simulink model "DualViennaRECT"  (R2021b)
settings: Solver=VariableStepAuto  StartTime=0.0  StopTime=1.5  RelTol=1e-3
libraries: spsIGBTDiodeLib x25, spsCurrentMeasurementLib x6, spsMeanLib x5, spsVoltageMeasurementLib x5, spsSeriesRLCBranchLib x3, spsMutualInductanceLib x3, spsACVoltageSourceLib x3, spsRMSLib x2, simulink x2, slpidlib x1, spsTHDLib x1, spspowerguiLib x1
settings Model: SimulationMode=accelerator  Creator=abc6820292  LastModifiedBy=abc6820292

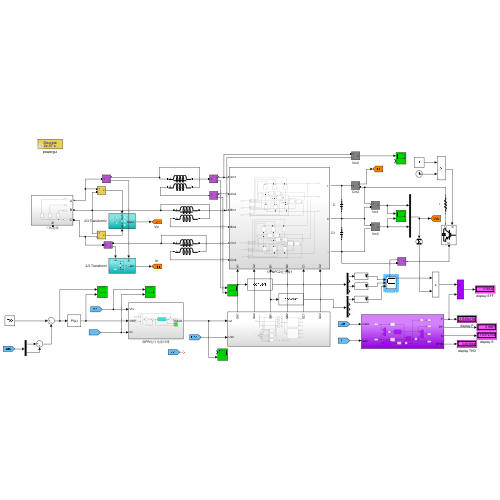
[thumbnail: Simulink's stored preview of the top-level diagram]
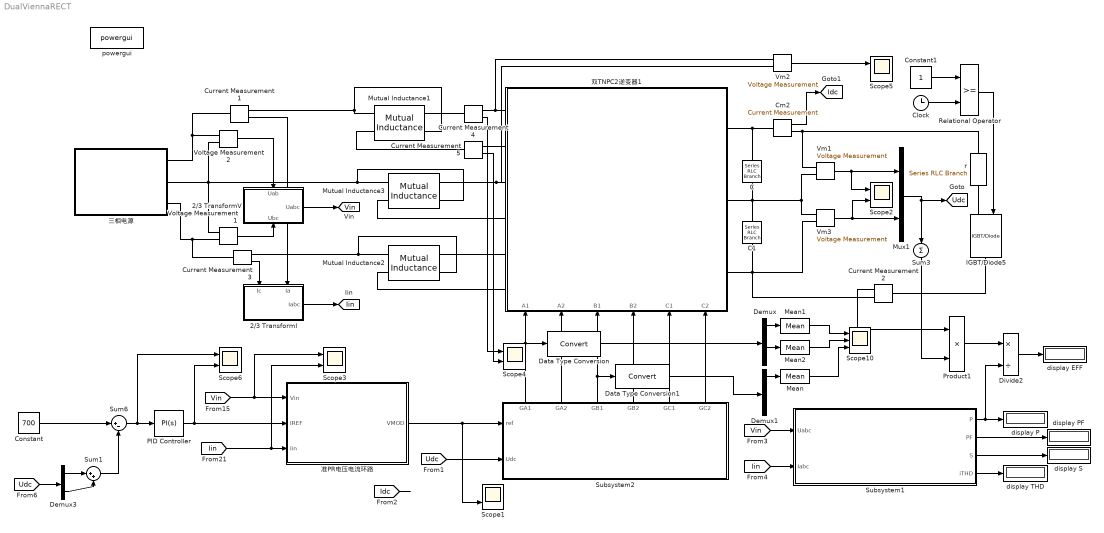
== system DualViennaRECT ==
  2/3 TransformI : Subsystem
      settings: PortSchema="{\"entries\":[{\"content\":{\"sides\":[{\"content\":{\"connectorIds\":[\"In1\",\"In2\"]},\"type\":\"ConnectorPlacement.EquallySpacedRectSide\",\"uuid\":\"58c40194-9a95-4e39-952e-f878bde7484e\"},{\"content\":{\"connectorIds\":[],\"side\":\"RIGHT\"},\"type\":\"ConnectorPlacement.EquallySpacedRectSide\",\"uuid\":\"f51692e8-3ff2-4d72-808d-3667196a4526\"},{\"content\":{\"connectorIds\":[],\"side\":\"TOP\"},\"type\":\"ConnectorPlacement.EquallySpacedRectSide\",\"uuid\":\"0aab136b-5da5-45c4-8998-999ebe8b7f2f\"},{\"content\":{\"connectorIds\":[\"Out1\"],\"side\":\"BOTTOM\"},\"type\":\"ConnectorPlacement.EquallySpacedRectSide\",\"uuid\":\"32f5f4a5-4ebb-496b-828d-b973bd46b44e\"}]},\"type\":\"ConnectorPlacement.EquallySpacedConnector\",\"uuid\":\"3ef81af7-d426-47fb-88e3-e33e58eebb83\"}],\"packageUris\":[\"http://schema.mathworks.com/mf0/Connector/R2020b\"],\"version\":\"1.0\"}"
  2/3 TransformV : Subsystem
      settings: PortSchema="{\"entries\":[{\"content\":{\"sides\":[{\"content\":{\"connectorIds\":[\"In1\"]},\"type\":\"ConnectorPlacement.EquallySpacedRectSide\",\"uuid\":\"58c40194-9a95-4e39-952e-f878bde7484e\"},{\"content\":{\"connectorIds\":[\"In2\"],\"side\":\"RIGHT\"},\"type\":\"ConnectorPlacement.EquallySpacedRectSide\",\"uuid\":\"f51692e8-3ff2-4d72-808d-3667196a4526\"},{\"content\":{\"connectorIds\":[],\"side\":\"TOP\"},\"type\":\"ConnectorPlacement.EquallySpacedRectSide\",\"uuid\":\"0aab136b-5da5-45c4-8998-999ebe8b7f2f\"},{\"content\":{\"connectorIds\":[\"Out1\"],\"side\":\"BOTTOM\"},\"type\":\"ConnectorPlacement.EquallySpacedRectSide\",\"uuid\":\"185ce796-68e2-4136-8080-97dc86d2ba54\"}]},\"type\":\"ConnectorPlacement.EquallySpacedConnector\",\"uuid\":\"3ef81af7-d426-47fb-88e3-e33e58eebb83\"}],\"packageUris\":[\"http://schema.mathworks.com/mf0/Connector/R2020b\"],\"version\":\"1.0\"}"
  C : spsSeriesRLCBranchLib/Series RLC Branch  LConnTagsString=__new0  RConnTagsString=__new0  BranchType=C  Resistance=0  Inductance=0  SetiL0=off  InitialCurrent=0  Capacitance=8e-3  Setx0=on  InitialVoltage=280  Measurements=None
  C1 : spsSeriesRLCBranchLib/Series RLC Branch  LConnTagsString=__new0  RConnTagsString=__new0  BranchType=C  Resistance=0  Inductance=0  SetiL0=off  InitialCurrent=0  Capacitance=8e-3  Setx0=on  InitialVoltage=280  Measurements=None
  Clock : Clock
  Cm2 : spsCurrentMeasurementLib/Current Measurement  PhasorSimulation=off  OutputType=Complex  PSBequivalent=0
  Constant : Constant  Value=700
  Constant1 : Constant
  Current Measurement{1..5} (5 alike) : spsCurrentMeasurementLib/Current Measurement  PhasorSimulation=off  OutputType=Complex  PSBequivalent=0
  Data Type Conversion : DataTypeConversion
  Data Type Conversion1 : DataTypeConversion
  Demux : Demux
  Demux1 : Demux
  Demux3 : Demux  Outputs=2
  Divide2 : Product  Inputs=*/
  IGBT/Diode5 : spsIGBTDiodeLib/IGBT//Diode  Ron=1e-3  Rs=1e5  Cs=inf  Measurements=off
  Mean : spsMeanLib/Mean  Freq=1000  Vinit=0  Ts=0
  Mean1 : spsMeanLib/Mean  Freq=1000  Vinit=0  Ts=0
  Mean2 : spsMeanLib/Mean  Freq=1000  Vinit=0  Ts=0
  Mutual Inductance1 : spsMutualInductanceLib/Mutual Inductance  LConnTagsString=a|b  RConnTagsString=A|B  TypeOfMutual=Two or three windings with equal mutual terms  NumberOfWindings=3  SelfImpedance1=[0.01 1e-3]  SelfImpedance2=[0.01 1e-3]  ThreeWindings=off  SelfImpedance3=[ 1.1 1.1e-03]  MutualImpedance=[0.05 6e-4]  InductanceMatrix="[1.0 0.9  0.9 ;  0.9 1.0  0.9;  0.9 0.9 1.0 ] * 1e-3"  ResistanceMatrix="[1.0 0.9  0.9 ;  0.9 1.0  0.9;  0.9 0.9 1.0 ]"  Measurements=None
      settings: SourceProductBaseCode=PS
  Mutual Inductance2 : spsMutualInductanceLib/Mutual Inductance  LConnTagsString=a|b  RConnTagsString=A|B  TypeOfMutual=Two or three windings with equal mutual terms  NumberOfWindings=3  SelfImpedance1=[0.01 1e-3]  SelfImpedance2=[0.01 1e-3]  ThreeWindings=off  SelfImpedance3=[ 1.1 1.1e-03]  MutualImpedance=[0.05 6e-4]  InductanceMatrix="[1.0 0.9  0.9 ;  0.9 1.0  0.9;  0.9 0.9 1.0 ] * 1e-3"  ResistanceMatrix="[1.0 0.9  0.9 ;  0.9 1.0  0.9;  0.9 0.9 1.0 ]"  Measurements=None
      settings: SourceProductBaseCode=PS
  Mutual Inductance3 : spsMutualInductanceLib/Mutual Inductance  LConnTagsString=a|b  RConnTagsString=A|B  TypeOfMutual=Two or three windings with equal mutual terms  NumberOfWindings=3  SelfImpedance1=[0.01 1e-3]  SelfImpedance2=[0.01 1e-3]  ThreeWindings=off  SelfImpedance3=[ 1.1 1.1e-03]  MutualImpedance=[0.05 6e-4]  InductanceMatrix="[1.0 0.9  0.9 ;  0.9 1.0  0.9;  0.9 0.9 1.0 ] * 1e-3"  ResistanceMatrix="[1.0 0.9  0.9 ;  0.9 1.0  0.9;  0.9 0.9 1.0 ]"  Measurements=None
      settings: SourceProductBaseCode=PS
  Mux1 : Mux  Inputs=2
  PID Controller : slpidlib/PID Controller  Controller=PI  Form=Parallel  TimeDomain=Continuous-time  UseExternalTs=off  SampleTime=-1  IntegratorMethod=Forward Euler  FilterMethod=Forward Euler  ControllerParametersSource=internal  P=0.3  I=6  D=0.001  UseFilter=on  N=100  TunerSelectOption=Transfer Function Based (PID Tuner App)  InitialConditionSource=internal  InitialConditionForIntegrator=0  InitialConditionForFilter=0  DifferentiatorICPrevScaledInput=0  ExternalReset=none  TrackingMode=off  Kt=1  LimitOutput=off  SatLimitsSource=internal  UpperSaturationLimit=100  LowerSaturationLimit=-100  LinearizeAsGain=on  AntiWindupMode=clamping  Kb=1  POutMin=[]  POutMax=[]  IOutMin=[]  IOutMax=[]  DOutMin=[]  DOutMax=[]  NOutMin=[]  NOutMax=[]  SumOutMin=[]  SumOutMax=[]  SaturationOutMin=[]  SaturationOutMax=[]  PParamMin=[]  PParamMax=[]  IParamMin=[]  IParamMax=[]  DParamMin=[]  DParamMax=[]  NParamMin=[]  NParamMax=[]  KbParamMin=[]  KbParamMax=[]  KtParamMin=[]  KtParamMax=[]  KbOutMin=[]  KbOutMax=[]  KtOutMin=[]  KtOutMax=[]  IntegratorOutMin=[]  IntegratorOutMax=[]  FilterOutMin=[]  FilterOutMax=[]  SumI1OutMin=[]  SumI1OutMax=[]  SumI2OutMin=[]  SumI2OutMax=[]  SumI3OutMin=[]  SumI3OutMax=[]  SumI4OutMin=[]  SumI4OutMax=[]  SumDOutMin=[]  SumDOutMax=[]  DifferentiatorOutMin=[]  DifferentiatorOutMax=[]  FilterDiffOutCoefMin=[]  FilterDiffOutCoefMax=[]  ReciprocalOutMin=[]  ReciprocalOutMax=[]  SumDenOutMin=[]  SumDenOutMax=[]  SumNumOutMin=[]  SumNumOutMax=[]  DivideOutMin=[]  DivideOutMax=[]  UdiffTsProdOutMin=[]  UdiffTsProdOutMax=[]  NTsProdOutMin=[]  NTsProdOutMax=[]  UintegralTsProdOutMin=[]  UintegralTsProdOutMax=[]  UngainTsProdOutMin=[]  UngainTsProdOutMax=[]  FilterDenConstantOutDataTypeStr=Inherit: Inherit via back propagation  FilterDenConstantOutMin=[]  FilterDenConstantOutMax=[]  PCopyOutDataTypeStr=Inherit: Inherit via back propagation  PCopyOutMin=[]  PCopyOutMax=[]  NCopyOutDataTypeStr=Inherit: Inherit via back propagation  NCopyOutMin=[]  NCopyOutMax=[]  IntegratorContinuousStateAttributes=''  IntegratorStateMustResolveToSignalObject=off  IntegratorRTWStateStorageClass=Auto  FilterContinuousStateAttributes=''  FilterStateMustResolveToSignalObject=off  FilterRTWStateStorageClass=Auto  ParallelPVariant=InternalParameters  IdealPVariant=Disabled  IVariant=InternalParameters  DVariant=Disabled  IntegratorVariant=Continuous  SatVariant=Disabled  AWVariant=Passthrough  PCopyVariant=Disabled  TRVariant=Disabled  FdbkBlocksVariant=Forward  IdealPFdbkVariant=Disabled  SatFdbkVariant=Disabled  DerivativeFilterVariant=Disabled  NVariant=Disabled  NCopyVariant=Disabled_SignalSpec  FilterICVariant=Disabled  IntegratorICVariant=InternalICs  ExternalResetVariant=Disabled  TRSumVariant=Passthrough  SumFdbkVariant=Disabled  SumVariant=Sum_PI  TsampFilterVariant=InternalTs  TsampNgainVariant=Passthrough  TsampIntegralVariant=Passthrough  ExternalSaturationOutDataTypeStr=Inherit: Same as second input
  Product1 : Product
  Relational Operator : RelationalOperator  OutDataTypeStr=boolean  RndMeth=Nearest
  Scope{1..6} (6 alike) : Scope  NumInputPorts=2
  Scope10 : Scope  NumInputPorts=3
  Subsystem1 : Subsystem
  Subsystem2 : Subsystem
      settings: PortSchema="{\"entries\":[{\"content\":{\"sides\":[{\"content\":{\"connectorIds\":[\"In1\",\"In2\"]},\"type\":\"ConnectorPlacement.EquallySpacedRectSide\",\"uuid\":\"86d8a801-af54-4615-919a-9a70996995f5\"},{\"content\":{\"connectorIds\":[],\"side\":\"RIGHT\"},\"type\":\"ConnectorPlacement.EquallySpacedRectSide\",\"uuid\":\"9c099dd5-197a-4a29-8cd5-6822de601230\"},{\"content\":{\"connectorIds\":[\"Out1\",\"Out2\",\"Out3\",\"Out4\",\"Out5\",\"Out6\"],\"side\":\"TOP\"},\"type\":\"ConnectorPlacement.EquallySpacedRectSide\",\"uuid\":\"5852d946-2383-4602-be71-32d16fa24bc3\"}]},\"type\":\"ConnectorPlacement.EquallySpacedConnector\",\"uuid\":\"a21c857f-e780-49b2-9a65-1676cf4540b1\"}],\"packageUris\":[\"http://schema.mathworks.com/mf0/Connector/R2020b\"],\"version\":\"1.0\"}"
  Sum1 : Sum  Inputs=|++
  Sum3 : Sum  Inputs=+
  Sum6 : Sum  Inputs=|+-
  Vm1 : spsVoltageMeasurementLib/Voltage Measurement  PhasorSimulation=off  OutputType=Complex  PSBequivalent=0
  Vm2 : spsVoltageMeasurementLib/Voltage Measurement  PhasorSimulation=off  OutputType=Complex  PSBequivalent=0
  Vm3 : spsVoltageMeasurementLib/Voltage Measurement  PhasorSimulation=off  OutputType=Complex  PSBequivalent=0
  Voltage Measurement1 : spsVoltageMeasurementLib/Voltage Measurement  PhasorSimulation=off  OutputType=Complex  PSBequivalent=0
  Voltage Measurement2 : spsVoltageMeasurementLib/Voltage Measurement  PhasorSimulation=off  OutputType=Complex  PSBequivalent=0
  display EFF : Display
  display P : Display
  display PF : Display
  display S : Display
  display THD : Display
  powergui : spspowerguiLib/powergui  SimulationMode=Discrete  SampleTime=2e-7  frequency=60  Iterations=50  frequencyindice=0  Pbase=100e6  ErrMax=1e-4  UnitsV=kV  UnitsW=MW  buscounter=0  FunctionMessages=off  echomessages=off  EnableUseOfTLC=off  CurrentSourceSwitches=off  DisableSnubberDevices=off  DisableRonSwitches=off  DisableVfSwitches=off  DisplayEquations=off  AutomaticDiscreteSolvers=off  SolverType=Tustin/Backward Euler (TBE)  Interpol=off  ExternalGateDelay=off  methode=off  Ts=0  x0status=blocks  SPID=off  SwTol=0  HookPort=off  NonlinearTolerance=1e-4  nMaxIteration=100  ContinueOnMaxIteration=off  RestoreLinks=warning  ResistiveCurrentMeasurement=off  Frange=[0:2:500]  Ylog=off  Xlog=on  ShowGrid=off  save=off  variable=ZData  structure=QQQQQ  ZoomFFT=off  StartTime=0.5  cycles=15  DisplayStyle=1  fundamental=50  FreqAxis=off  MaxFrequency=1000  frequencyindicesteady=1  RmsSteady=1  display=off
  r : spsSeriesRLCBranchLib/Series RLC Branch  LConnTagsString=__new0  RConnTagsString=__new0  BranchType=R  Resistance=30  Inductance=12e-4  SetiL0=off  InitialCurrent=0  Capacitance=inf  Setx0=off  InitialVoltage=0  Measurements=None
  三相电源 : Subsystem
      settings: PortSchema="{\"entries\":[{\"content\":{\"sides\":[{\"content\":{\"connectorIds\":[]},\"type\":\"ConnectorPlacement.EquallySpacedRectSide\",\"uuid\":\"5692784f-1b55-4d91-979b-6d4f0f069822\"},{\"content\":{\"connectorIds\":[\"RConn1\",\"RConn2\",\"RConn3\"],\"side\":\"RIGHT\"},\"type\":\"ConnectorPlacement.EquallySpacedRectSide\",\"uuid\":\"9a030936-b32a-4f05-b3f8-cc4c8aa25605\"},{\"content\":{\"connectorIds\":[],\"side\":\"TOP\"},\"type\":\"ConnectorPlacement.EquallySpacedRectSide\",\"uuid\":\"5cfc997e-60a4-43d8-bb4b-1dd6701aa9aa\"},{\"content\":{\"connectorIds\":[\"RConn4\"],\"side\":\"BOTTOM\"},\"type\":\"ConnectorPlacement.EquallySpacedRectSide\",\"uuid\":\"c52a786f-991d-42ea-bd6e-73a9c9371acb\"}]},\"type\":\"ConnectorPlacement.EquallySpacedConnector\",\"uuid\":\"853efb3d-2dc6-42ad-992e-f1defcaa0d46\"}],\"packageUris\":[\"http://schema.mathworks.com/mf0/Connector/R2020b\"],\"version\":\"1.0\"}"
  准PR电压电流环路 : Subsystem
  双TNPC2逆变器1 : Subsystem
      settings: PortSchema="{\"entries\":[{\"content\":{\"sides\":[{\"content\":{\"connectorIds\":[\"LConn1\",\"LConn2\",\"LConn3\",\"LConn4\",\"LConn5\",\"LConn6\"]},\"type\":\"ConnectorPlacement.EquallySpacedRectSide\",\"uuid\":\"47187a24-6853-42ac-9ad9-0df0e1360fae\"},{\"content\":{\"connectorIds\":[\"RConn1\",\"RConn2\",\"RConn3\"],\"side\":\"RIGHT\"},\"type\":\"ConnectorPlacement.EquallySpacedRectSide\",\"uuid\":\"b3504369-b235-4116-9b9b-167bd6b76527\"},{\"content\":{\"connectorIds\":[],\"side\":\"TOP\"},\"type\":\"ConnectorPlacement.EquallySpacedRectSide\",\"uuid\":\"5cb205b4-da18-4f20-b3d4-22846a9c2236\"},{\"content\":{\"connectorIds\":[\"In1\",\"In2\",\"In3\",\"In4\",\"In5\",\"In6\"],\"side\":\"BOTTOM\"},\"type\":\"ConnectorPlacement.EquallySpacedRectSide\",\"uuid\":\"4e548a82-6bdf-470e-8572-00c7c8855d01\"}]},\"type\":\"ConnectorPlacement.EquallySpacedConnector\",\"uuid\":\"b00ba750-ea4b-4b64-a122-5cbc9e899126\"}],\"packageUris\":[\"http://schema.mathworks.com/mf0/Connector/R2020b\"],\"version\":\"1.0\"}"
  tag scope: Idc=global, Iin=global, Udc=global, Vin=global
  wires:
  Vm3/1 -> Scope2/2, Mux1/2
  Sum6/1 -> PID Controller/1, Scope6/1
  Constant/1 -> Sum6/1
  [Vin] -> 准PR电压电流环路/1(Vin), Scope3/1
  [Iin] -> 准PR电压电流环路/3(Iin), Scope3/2
  准PR电压电流环路/1(VMOD) -> Scope1/2, Subsystem2/1(ref)
  Subsystem2/1(GA1) -> 双TNPC2逆变器1/1(A1), Data Type Conversion/1
  Subsystem2/3(GB1) -> Data Type Conversion1/1, 双TNPC2逆变器1/3(B1)
  Subsystem2/5(GC1) -> 双TNPC2逆变器1/5(C1)
  Vm1/1 -> Scope2/1, Mux1/1
  Mux1/1 -> Sum3/1, [Udc]
  [Udc] -> Demux3/1
  Demux3/1 -> Sum1/1
  Demux3/2 -> Sum1/2
  Sum1/1 -> Sum6/2
  Cm2/1 -> [Idc]
  Vm2/1 -> Scope5/1
  [Vin] -> Subsystem1/1(Uabc)
  [Iin] -> Subsystem1/2(Iabc)
  PID Controller/1 -> 准PR电压电流环路/2(IREF), Scope6/2
  Subsystem1/1(P) -> Divide2/2, display P/1
  Subsystem1/2(PF) -> display PF/1
  Subsystem1/4(iTHD) -> display THD/1
  Subsystem1/3(S) -> display S/1
  Current Measurement2/1 -> Product1/1
  Sum3/1 -> Product1/2
  Product1/1 -> Divide2/1
  Divide2/1 -> display EFF/1
  Voltage Measurement1/1 -> 2/3 TransformV/2(Ubc)
  Voltage Measurement2/1 -> 2/3 TransformV/1(Uab)
  2/3 TransformV/1(Uabc) -> [Vin]
  Current Measurement3/1 -> 2/3 TransformI/1(Ic)
  Current Measurement1/1 -> 2/3 TransformI/2(Ia)
  2/3 TransformI/1(Iabc) -> [Iin]
  Subsystem2/2(GA2) -> 双TNPC2逆变器1/2(A2)
  Subsystem2/4(GB2) -> 双TNPC2逆变器1/4(B2)
  Subsystem2/6(GC2) -> 双TNPC2逆变器1/6(C2)
  Mean1/1 -> Scope10/1
  Demux/1 -> Mean1/1
  Mean/1 -> Scope10/3
  Demux/3 -> Mean2/1
  Demux1/1 -> Mean/1
  Mean2/1 -> Scope10/2
  Data Type Conversion/1 -> Demux/1
  Data Type Conversion1/1 -> Demux1/1
  Current Measurement4/1 -> Scope4/1
  Current Measurement5/1 -> Scope4/2
  Constant1/1 -> Relational Operator/1
  Clock/1 -> Relational Operator/2
  Relational Operator/1 -> IGBT/Diode5/1
  [Udc] -> Subsystem2/2(Udc)
  [Idc] -> ?
  connections:
  三相电源/RConn2 -- Voltage Measurement1/LConn1 -- Voltage Measurement2/LConn2 -- Mutual Inductance3/RConn2 -- Mutual Inductance3/LConn1
  Mutual Inductance2/RConn2 -- Current Measurement3/RConn1 -- Mutual Inductance2/LConn1
  Vm1/LConn1 -- r/LConn1 -- Cm2/RConn1
  C/RConn1 -- 双TNPC2逆变器1/RConn2 -- Vm3/LConn1 -- Vm1/LConn2 -- C1/LConn1
  C1/RConn1 -- 双TNPC2逆变器1/RConn3 -- Current Measurement2/RConn1 -- Vm3/LConn2
  C/LConn1 -- 双TNPC2逆变器1/RConn1 -- Cm2/LConn1
  三相电源/RConn1 -- Voltage Measurement2/LConn1 -- Current Measurement1/LConn1
  Voltage Measurement1/LConn2 -- 三相电源/RConn3 -- Current Measurement3/LConn1
  双TNPC2逆变器1/LConn5 -- Mutual Inductance2/RConn1
  双TNPC2逆变器1/LConn3 -- Vm2/LConn2 -- Mutual Inductance3/RConn1
  双TNPC2逆变器1/LConn4 -- Mutual Inductance3/LConn2
  双TNPC2逆变器1/LConn6 -- Mutual Inductance2/LConn2
  Current Measurement4/LConn1 -- Mutual Inductance1/RConn1
  双TNPC2逆变器1/LConn1 -- Vm2/LConn1 -- Current Measurement4/RConn1
  Mutual Inductance1/LConn1 -- Current Measurement1/RConn1 -- Mutual Inductance1/RConn2
  双TNPC2逆变器1/LConn2 -- Current Measurement5/RConn1
  Current Measurement5/LConn1 -- Mutual Inductance1/LConn2
  IGBT/Diode5/LConn1 -- r/RConn1
  IGBT/Diode5/RConn1 -- Current Measurement2/LConn1

== system DualViennaRECT/2//3 TransformI ==
  Ic : Inport
  Ia : Inport  Port=2
  Mux : Mux  Inputs=3
  Sum1 : Sum  Inputs=-|-
  Iabc : Outport
  wires:
  Ia/1 -> Sum1/1, Mux/1
  Ic/1 -> Sum1/2, Mux/3
  Mux/1 -> Iabc/1
  Sum1/1 -> Mux/2

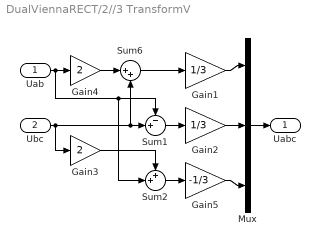
== system DualViennaRECT/2//3 TransformV ==
  Uab : Inport
  Ubc : Inport  Port=2
  Gain1 : Gain  Gain=1/3
  Gain2 : Gain  Gain=1/3
  Gain3 : Gain  Gain=2
  Gain4 : Gain  Gain=2
  Gain5 : Gain  Gain=-1/3
  Mux : Mux  Inputs=3
  Sum1 : Sum  Inputs=-+|
  Sum2 : Sum  Inputs=++|
  Sum6 : Sum  Inputs=|++
  Uabc : Outport
  wires:
  Sum6/1 -> Gain1/1
  Uab/1 -> Sum2/2, Sum1/1, Gain4/1
  Gain4/1 -> Sum6/1
  Ubc/1 -> Sum1/2, Sum6/2, Gain3/1
  Sum1/1 -> Gain2/1
  Gain3/1 -> Sum2/1
  Sum2/1 -> Gain5/1
  Gain2/1 -> Mux/2
  Gain5/1 -> Mux/3
  Gain1/1 -> Mux/1
  Mux/1 -> Uabc/1

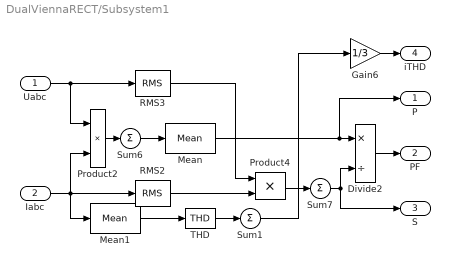
== system DualViennaRECT/Subsystem1 ==
  Uabc : Inport
  Iabc : Inport  Port=2
  Divide2 : Product  Inputs=*/
  Gain6 : Gain  Gain=1/3
  Mean : spsMeanLib/Mean  Freq=100  Vinit=0  Ts=0
  Mean1 : spsMeanLib/Mean  Freq=20000  Vinit=0  Ts=0
  Product2 : Product
  Product4 : Product
  RMS2 : spsRMSLib/RMS  TrueRMS=on  Freq=50  RMSInit=0  Ts=0
  RMS3 : spsRMSLib/RMS  TrueRMS=on  Freq=50  RMSInit=0  Ts=0
  Sum1 : Sum  Inputs=+
  Sum6 : Sum  Inputs=+
  Sum7 : Sum  Inputs=+
  THD : spsTHDLib/THD  Freq=50  Ts=0
      settings: SourceProductBaseCode=PS
  P : Outport
  PF : Outport  Port=2
  S : Outport  Port=3
  iTHD : Outport  Port=4
  wires:
  RMS3/1 -> Product4/1
  Product4/1 -> Sum7/1
  Sum6/1 -> Mean/1
  Product2/1 -> Sum6/1
  Divide2/1 -> PF/1
  RMS2/1 -> Product4/2
  Sum1/1 -> Gain6/1
  Gain6/1 -> iTHD/1
  Uabc/1 -> RMS3/1, Product2/1
  Sum7/1 -> S/1, Divide2/2
  Mean/1 -> P/1, Divide2/1
  Iabc/1 -> Mean1/1, Product2/2, RMS2/1
  THD/1 -> Sum1/1
  Mean1/1 -> THD/1

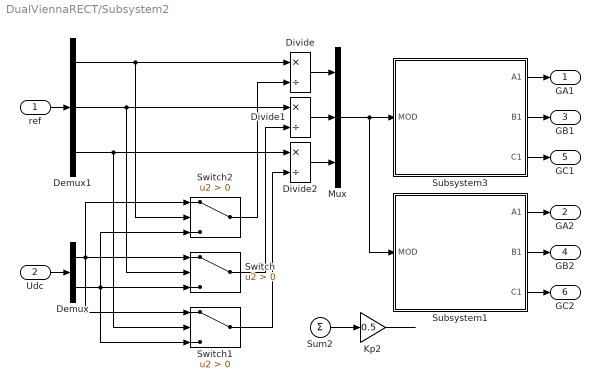
== system DualViennaRECT/Subsystem2 ==
  ref : Inport
  Udc : Inport  Port=2
  Demux : Demux  Outputs=2
  Demux1 : Demux  Outputs=3
  Divide : Product  Inputs=*/
  Divide1 : Product  Inputs=*/
  Divide2 : Product  Inputs=*/
  Kp2 : Gain  Gain=0.5
  Mux : Mux  Inputs=3
  Subsystem1 : Subsystem
  Subsystem3 : Subsystem
  Sum2 : Sum  Inputs=+
  Switch : Switch  Criteria=u2 > Threshold
  Switch1 : Switch  Criteria=u2 > Threshold
  Switch2 : Switch  Criteria=u2 > Threshold
  GA1 : Outport
  GA2 : Outport  Port=2
  GB1 : Outport  Port=3
  GB2 : Outport  Port=4
  GC1 : Outport  Port=5
  GC2 : Outport  Port=6
  wires:
  Subsystem3/1(A1) -> GA1/1
  Kp2/1 -> ?
  Subsystem3/2(B1) -> GB1/1
  Subsystem3/3(C1) -> GC1/1
  Subsystem1/2(B1) -> GB2/1
  Subsystem1/1(A1) -> GA2/1
  Subsystem1/3(C1) -> GC2/1
  Mux/1 -> Subsystem1/1(MOD), Subsystem3/1(MOD)
  Sum2/1 -> Kp2/1
  Udc/1 -> Demux/1
  ref/1 -> Demux1/1
  Demux1/2 -> Divide1/1, Switch/2
  Demux1/3 -> Divide2/1, Switch1/2
  Demux/2 -> Switch1/3, Switch2/3, Switch/3
  Demux/1 -> Switch2/1, Switch1/1, Switch/1
  Demux1/1 -> Switch2/2, Divide/1
  Switch2/1 -> Divide/2
  Switch/1 -> Divide1/2
  Switch1/1 -> Divide2/2
  Divide1/1 -> Mux/2
  Divide/1 -> Mux/1
  Divide2/1 -> Mux/3

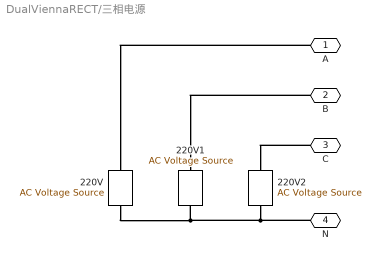
== system DualViennaRECT/三相电源 ==
  220V : spsACVoltageSourceLib/AC Voltage Source  Amplitude=310  Phase=0  Frequency=50  SampleTime=0  Measurements=None  BusType=swing  Pref=10e3  Qref=0  Qmin=-inf  Qmax=+inf
  220V1 : spsACVoltageSourceLib/AC Voltage Source  Amplitude=310  Phase=120  Frequency=50  SampleTime=0  Measurements=None  BusType=swing  Pref=10e3  Qref=0  Qmin=-inf  Qmax=+inf
  220V2 : spsACVoltageSourceLib/AC Voltage Source  Amplitude=310  Phase=-120  Frequency=50  SampleTime=0  Measurements=None  BusType=swing  Pref=10e3  Qref=0  Qmin=-inf  Qmax=+inf
  A : PMIOPort  Side=Right
  B : PMIOPort  Port=2  Side=Right
  C : PMIOPort  Port=3  Side=Right
  N : PMIOPort  Port=4  Side=Right
  connections:
  220V/LConn1 -- N/RConn1 -- 220V2/LConn1 -- 220V1/LConn1
  A/RConn1 -- 220V/RConn1
  B/RConn1 -- 220V1/RConn1
  C/RConn1 -- 220V2/RConn1

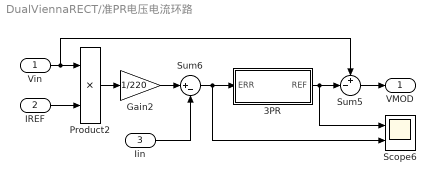
== system DualViennaRECT/准PR电压电流环路 ==
  Vin : Inport
  IREF : Inport  Port=2
  Iin : Inport  Port=3
  3PR : Subsystem
      settings: PortSchema="{\"entries\":[{\"content\":{\"sides\":[{\"content\":{\"connectorIds\":[]},\"type\":\"ConnectorPlacement.EquallySpacedRectSide\",\"uuid\":\"ac756fcf-f6d7-466d-bb3d-287dec8ae983\"},{\"content\":{\"connectorIds\":[],\"side\":\"RIGHT\"},\"type\":\"ConnectorPlacement.EquallySpacedRectSide\",\"uuid\":\"3e1a0e91-a0b8-40c4-8839-5ebd84050a30\"},{\"content\":{\"connectorIds\":[\"In1\"],\"side\":\"TOP\"},\"type\":\"ConnectorPlacement.EquallySpacedRectSide\",\"uuid\":\"4c3986ff-483b-4975-8d50-1a8a46f35065\"},{\"content\":{\"connectorIds\":[\"Out1\"],\"side\":\"BOTTOM\"},\"type\":\"ConnectorPlacement.EquallySpacedRectSide\",\"uuid\":\"d0166e46-df65-4061-a961-140d500477a7\"}]},\"type\":\"ConnectorPlacement.EquallySpacedConnector\",\"uuid\":\"9d4b00aa-dfb1-427d-8698-7ec64c5ca012\"}],\"packageUris\":[\"http://schema.mathworks.com/mf0/Connector/R2020b\"],\"version\":\"1.0\"}"
  Gain2 : Gain  Gain=1/220
  Product2 : Product
  Scope6 : Scope  NumInputPorts=2
  Sum5 : Sum  Inputs=+-|
  Sum6 : Sum  Inputs=|+-
  VMOD : Outport
  wires:
  IREF/1 -> Product2/2
  Sum5/1 -> VMOD/1
  Sum6/1 -> Scope6/2, 3PR/1(ERR)
  Product2/1 -> Gain2/1
  Iin/1 -> Sum6/2
  3PR/1(REF) -> Scope6/1, Sum5/2
  Gain2/1 -> Sum6/1
  Vin/1 -> Product2/1, Sum5/1

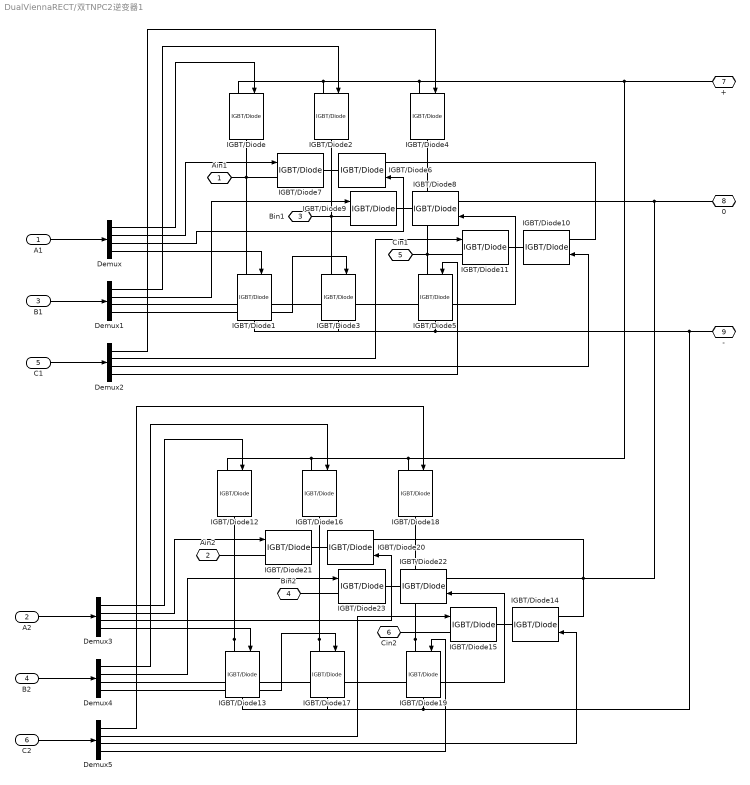
== system DualViennaRECT/双TNPC2逆变器1 ==
  A1 : Inport
  A2 : Inport  Port=2
  B1 : Inport  Port=3
  B2 : Inport  Port=4
  C1 : Inport  Port=5
  C2 : Inport  Port=6
  Demux{,1..5} (6 alike) : Demux
  IGBT/Diode{,1..23} (24 alike) : spsIGBTDiodeLib/IGBT//Diode  Ron=1e-3  Rs=1e5  Cs=inf  Measurements=off
  Ain1 : PMIOPort  Side=Left
  Ain2 : PMIOPort  Port=2  Side=Left
  Bin1 : PMIOPort  Port=3  Side=Left
  Bin2 : PMIOPort  Port=4  Side=Left
  Cin1 : PMIOPort  Port=5  Side=Left
  Cin2 : PMIOPort  Port=6  Side=Left
  + : PMIOPort  Port=7  Side=Right
  0 : PMIOPort  Port=8  Side=Right
  - : PMIOPort  Port=9  Side=Right
  wires:
  Demux/1 -> IGBT/Diode/1
  A1/1 -> Demux/1
  Demux1/1 -> IGBT/Diode2/1
  Demux2/1 -> IGBT/Diode4/1
  B1/1 -> Demux1/1
  C1/1 -> Demux2/1
  Demux2/4 -> IGBT/Diode5/1
  Demux1/4 -> IGBT/Diode3/1
  Demux/4 -> IGBT/Diode1/1
  Demux3/4 -> IGBT/Diode13/1
  B2/1 -> Demux4/1
  C2/1 -> Demux5/1
  Demux3/1 -> IGBT/Diode12/1
  Demux5/4 -> IGBT/Diode19/1
  Demux4/1 -> IGBT/Diode16/1
  A2/1 -> Demux3/1
  Demux4/4 -> IGBT/Diode17/1
  Demux5/1 -> IGBT/Diode18/1
  Demux/2 -> IGBT/Diode7/1
  Demux/3 -> IGBT/Diode6/1
  Demux1/2 -> IGBT/Diode9/1
  Demux1/3 -> IGBT/Diode8/1
  Demux2/2 -> IGBT/Diode11/1
  Demux2/3 -> IGBT/Diode10/1
  Demux3/2 -> IGBT/Diode21/1
  Demux3/3 -> IGBT/Diode20/1
  Demux4/2 -> IGBT/Diode23/1
  Demux4/3 -> IGBT/Diode22/1
  Demux5/2 -> IGBT/Diode15/1
  Demux5/3 -> IGBT/Diode14/1
  connections:
  IGBT/Diode2/RConn1 -- IGBT/Diode9/LConn1 -- Bin1/RConn1 -- IGBT/Diode3/LConn1
  IGBT/Diode18/LConn1 -- IGBT/Diode/LConn1 -- IGBT/Diode2/LConn1 -- IGBT/Diode4/LConn1 -- +/RConn1 -- IGBT/Diode12/LConn1 -- IGBT/Diode16/LConn1
  IGBT/Diode4/RConn1 -- Cin1/RConn1 -- IGBT/Diode11/LConn1 -- IGBT/Diode5/LConn1
  IGBT/Diode19/RConn1 -- IGBT/Diode1/RConn1 -- IGBT/Diode3/RConn1 -- IGBT/Diode5/RConn1 -- -/RConn1 -- IGBT/Diode13/RConn1 -- IGBT/Diode17/RConn1
  IGBT/Diode/RConn1 -- Ain1/RConn1 -- IGBT/Diode7/LConn1 -- IGBT/Diode1/LConn1
  IGBT/Diode7/RConn1 -- IGBT/Diode6/RConn1
  IGBT/Diode20/LConn1 -- 0/RConn1 -- IGBT/Diode10/LConn1 -- IGBT/Diode8/LConn1 -- IGBT/Diode6/LConn1 -- IGBT/Diode14/LConn1 -- IGBT/Diode22/LConn1
  IGBT/Diode9/RConn1 -- IGBT/Diode8/RConn1
  IGBT/Diode11/RConn1 -- IGBT/Diode10/RConn1
  IGBT/Diode19/LConn1 -- IGBT/Diode18/RConn1 -- Cin2/RConn1 -- IGBT/Diode15/LConn1
  IGBT/Diode13/LConn1 -- IGBT/Diode12/RConn1 -- Ain2/RConn1 -- IGBT/Diode21/LConn1
  IGBT/Diode17/LConn1 -- IGBT/Diode16/RConn1 -- IGBT/Diode23/LConn1 -- Bin2/RConn1
  IGBT/Diode23/RConn1 -- IGBT/Diode22/RConn1
  IGBT/Diode21/RConn1 -- IGBT/Diode20/RConn1
  IGBT/Diode15/RConn1 -- IGBT/Diode14/RConn1

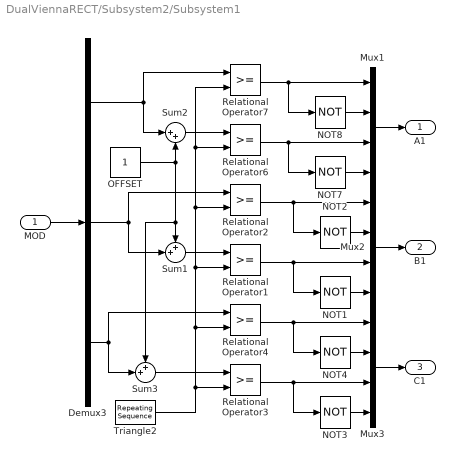
== system DualViennaRECT/Subsystem2/Subsystem1 ==
  MOD : Inport
  Demux3 : Demux  Outputs=3
  Mux1 : Mux
  Mux2 : Mux
  Mux3 : Mux
  NOT{1..4,7..8} (6 alike) : Logic  Operator=NOT  IconShape=distinctive  AllPortsSameDT=off  OutDataTypeStr=boolean
  OFFSET : Constant
  Relational Operator{1..4,6..7} (6 alike) : RelationalOperator  OutDataTypeStr=boolean  RndMeth=Nearest
  Sum1 : Sum  Inputs=++|
  Sum2 : Sum  Inputs=|++
  Sum3 : Sum  Inputs=++|
  Triangle2 : simulink/Sources/Repeating Sequence  rep_seq_t=[0 1/20000/2 1/20000]  rep_seq_y=[1 0 1]
  A1 : Outport
  B1 : Outport  Port=2
  C1 : Outport  Port=3
  wires:
  Demux3/3 -> Sum3/2, Relational Operator4/1
  Sum3/1 -> Relational Operator3/1
  Sum1/1 -> Relational Operator1/1
  Demux3/2 -> Sum1/2, Relational Operator2/1
  Relational Operator4/1 -> NOT4/1, Mux3/1
  Relational Operator3/1 -> NOT3/1, Mux3/3
  NOT4/1 -> Mux3/2
  NOT3/1 -> Mux3/4
  NOT1/1 -> Mux2/4
  NOT2/1 -> Mux2/2
  Relational Operator1/1 -> Mux2/3, NOT1/1
  Relational Operator2/1 -> NOT2/1, Mux2/1
  Demux3/1 -> Relational Operator7/1, Sum2/1
  NOT8/1 -> Mux1/2
  Triangle2/1 -> Relational Operator6/2, Relational Operator7/2, Relational Operator2/2, Relational Operator1/2, Relational Operator4/2, Relational Operator3/2
  Relational Operator7/1 -> NOT8/1, Mux1/1
  NOT7/1 -> Mux1/4
  Sum2/1 -> Relational Operator6/1
  Relational Operator6/1 -> Mux1/3, NOT7/1
  OFFSET/1 -> Sum2/2, Sum1/1, Sum3/1
  Mux2/1 -> B1/1
  Mux3/1 -> C1/1
  Mux1/1 -> A1/1
  MOD/1 -> Demux3/1

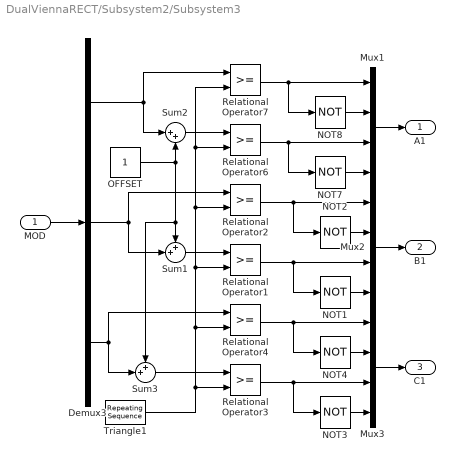
== system DualViennaRECT/Subsystem2/Subsystem3 ==
  MOD : Inport
  Demux3 : Demux  Outputs=3
  Mux1 : Mux
  Mux2 : Mux
  Mux3 : Mux
  NOT{1..4,7..8} (6 alike) : Logic  Operator=NOT  IconShape=distinctive  AllPortsSameDT=off  OutDataTypeStr=boolean
  OFFSET : Constant
  Relational Operator{1..4,6..7} (6 alike) : RelationalOperator  OutDataTypeStr=boolean  RndMeth=Nearest
  Sum1 : Sum  Inputs=++|
  Sum2 : Sum  Inputs=|++
  Sum3 : Sum  Inputs=++|
  Triangle1 : simulink/Sources/Repeating Sequence  rep_seq_t=[0 1/20000/2 1/20000]  rep_seq_y=[0 1 0]
  A1 : Outport
  B1 : Outport  Port=2
  C1 : Outport  Port=3
  wires:
  MOD/1 -> Demux3/1
  Mux1/1 -> A1/1
  Mux3/1 -> C1/1
  Mux2/1 -> B1/1
  OFFSET/1 -> Sum3/1, Sum1/1, Sum2/2
  Relational Operator6/1 -> NOT7/1, Mux1/3
  Sum2/1 -> Relational Operator6/1
  NOT7/1 -> Mux1/4
  Relational Operator7/1 -> Mux1/1, NOT8/1
  Triangle1/1 -> Relational Operator3/2, Relational Operator4/2, Relational Operator1/2, Relational Operator2/2, Relational Operator7/2, Relational Operator6/2
  NOT8/1 -> Mux1/2
  Demux3/1 -> Sum2/1, Relational Operator7/1
  Relational Operator2/1 -> Mux2/1, NOT2/1
  Relational Operator1/1 -> NOT1/1, Mux2/3
  NOT2/1 -> Mux2/2
  NOT1/1 -> Mux2/4
  NOT3/1 -> Mux3/4
  NOT4/1 -> Mux3/2
  Relational Operator3/1 -> Mux3/3, NOT3/1
  Relational Operator4/1 -> Mux3/1, NOT4/1
  Demux3/2 -> Relational Operator2/1, Sum1/2
  Sum1/1 -> Relational Operator1/1
  Sum3/1 -> Relational Operator3/1
  Demux3/3 -> Relational Operator4/1, Sum3/2

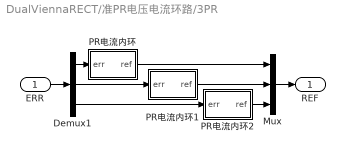
== system DualViennaRECT/准PR电压电流环路/3PR ==
  ERR : Inport
  Demux1 : Demux  Outputs=3
  Mux : Mux  Inputs=3
  PR电流内环 : Subsystem  TreatAsAtomicUnit=on  mask{Kp=1, Kr=80, Wc=5, Upper=80, Lower=-80}
  PR电流内环1 : Subsystem  TreatAsAtomicUnit=on  mask{Kp=1, Kr=80, Wc=5, Upper=80, Lower=-80}
  PR电流内环2 : Subsystem  TreatAsAtomicUnit=on  mask{Kp=1, Kr=80, Wc=5, Upper=80, Lower=-80}
  REF : Outport
  wires:
  ERR/1 -> Demux1/1
  Demux1/1 -> PR电流内环/1(err)
  Demux1/2 -> PR电流内环1/1(err)
  Demux1/3 -> PR电流内环2/1(err)
  PR电流内环2/1(ref) -> Mux/3
  PR电流内环/1(ref) -> Mux/1
  PR电流内环1/1(ref) -> Mux/2
  Mux/1 -> REF/1

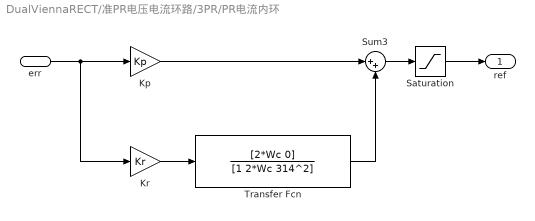
== system DualViennaRECT/准PR电压电流环路/3PR/PR电流内环 ==
  err : Inport
  Kp : Gain  Gain=Kp
  Kr : Gain  Gain=Kr
  Saturation : Saturate  UpperLimit=Upper  LowerLimit=Lower
  Sum3 : Sum  Inputs=|++
  Transfer Fcn : TransferFcn  Numerator=[2*Wc 0]  Denominator=[1 2*Wc 314^2]
  ref : Outport
  wires:
  Kp/1 -> Sum3/1
  Sum3/1 -> Saturation/1
  err/1 -> Kr/1, Kp/1
  Kr/1 -> Transfer Fcn/1
  Transfer Fcn/1 -> Sum3/2
  Saturation/1 -> ref/1

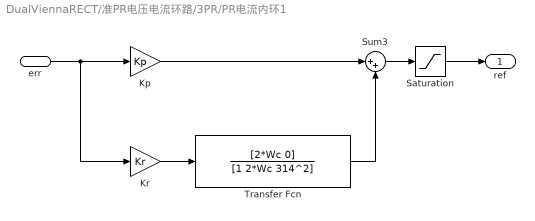
== system DualViennaRECT/准PR电压电流环路/3PR/PR电流内环1 ==
  err : Inport
  Kp : Gain  Gain=Kp
  Kr : Gain  Gain=Kr
  Saturation : Saturate  UpperLimit=Upper  LowerLimit=Lower
  Sum3 : Sum  Inputs=|++
  Transfer Fcn : TransferFcn  Numerator=[2*Wc 0]  Denominator=[1 2*Wc 314^2]
  ref : Outport
  wires:
  Kp/1 -> Sum3/1
  Sum3/1 -> Saturation/1
  err/1 -> Kr/1, Kp/1
  Kr/1 -> Transfer Fcn/1
  Transfer Fcn/1 -> Sum3/2
  Saturation/1 -> ref/1

== system DualViennaRECT/准PR电压电流环路/3PR/PR电流内环2 ==
  err : Inport
  Kp : Gain  Gain=Kp
  Kr : Gain  Gain=Kr
  Saturation : Saturate  UpperLimit=Upper  LowerLimit=Lower
  Sum3 : Sum  Inputs=|++
  Transfer Fcn : TransferFcn  Numerator=[2*Wc 0]  Denominator=[1 2*Wc 314^2]
  ref : Outport
  wires:
  Kp/1 -> Sum3/1
  Sum3/1 -> Saturation/1
  err/1 -> Kr/1, Kp/1
  Kr/1 -> Transfer Fcn/1
  Transfer Fcn/1 -> Sum3/2
  Saturation/1 -> ref/1
